simulink model "untitled2"  (R2022b)
settings: Solver=FixedStepAuto  StartTime=0  StopTime=1500  FixedStep=0.01  RelTol=1e-3
undefined symbols (not defined in the file or in its folder): sigbuilder_block
libraries: slpidlib x2
settings Model: Creator=hp  LastModifiedBy=hp

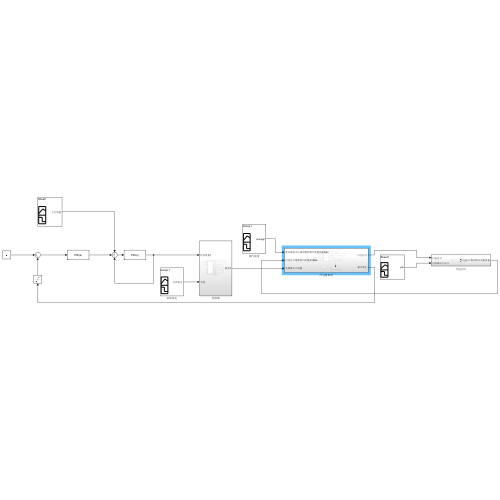
[thumbnail: Simulink's stored preview of the top-level diagram]
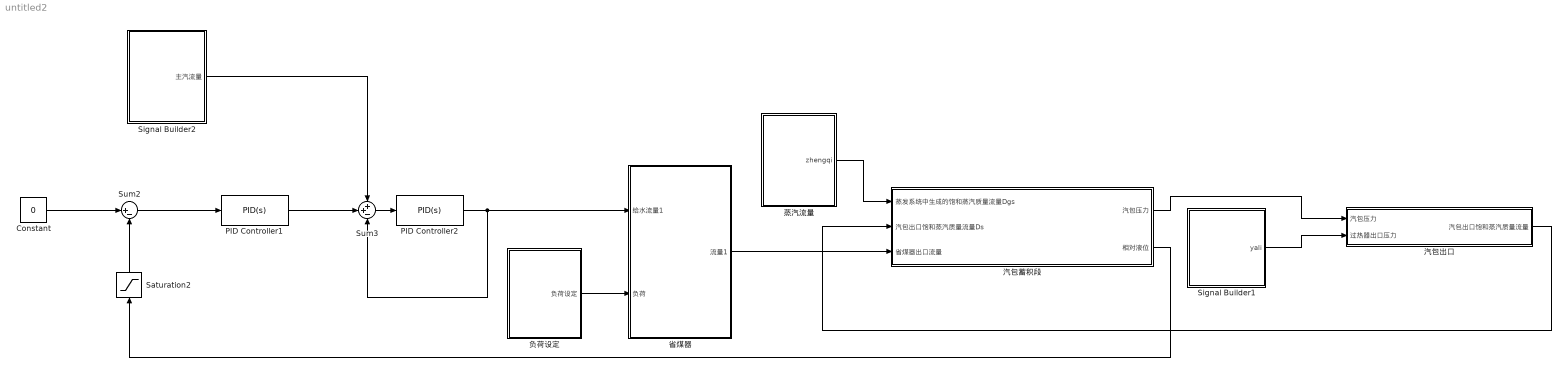
== system untitled2 ==
  Constant : Constant  Value=0
  PID Controller1 : slpidlib/PID Controller  Controller=PID  Form=Parallel  TimeDomain=Continuous-time  UseExternalTs=off  SampleTime=-1  IntegratorMethod=Forward Euler  FilterMethod=Forward Euler  ControllerParametersSource=internal  P=203.8263761763  I=22.4302136842899  UseKiTs=off  D=314.119346774621  N=0.810831032432681  UseFilter=on  TunerSelectOption=Transfer Function Based (PID Tuner App)  InitialConditionSource=internal  InitialConditionForIntegrator=0  InitialConditionForFilter=0  DifferentiatorICPrevScaledInput=0  ExternalReset=none  TrackingMode=off  Kt=1  LimitOutput=off  SatLimitsSource=internal  UpperSaturationLimit=inf  LowerSaturationLimit=-inf  LinearizeAsGain=on  AntiWindupMode=none  Kb=1  LimitIntegrator=off  UpperIntegratorSaturationLimit=inf  LowerIntegratorSaturationLimit=-inf  POutMin=[]  POutMax=[]  IOutMin=[]  IOutMax=[]  DOutMin=[]  DOutMax=[]  NOutMin=[]  NOutMax=[]  SumOutMin=[]  SumOutMax=[]  SaturationOutMin=[]  SaturationOutMax=[]  PParamMin=[]  PParamMax=[]  IParamMin=[]  IParamMax=[]  DParamMin=[]  DParamMax=[]  NParamMin=[]  NParamMax=[]  KbParamMin=[]  KbParamMax=[]  KtParamMin=[]  KtParamMax=[]  KbOutMin=[]  KbOutMax=[]  KtOutMin=[]  KtOutMax=[]  IntegratorOutMin=[]  IntegratorOutMax=[]  FilterOutMin=[]  FilterOutMax=[]  SumI1OutMin=[]  SumI1OutMax=[]  SumI2OutMin=[]  SumI2OutMax=[]  SumI3OutMin=[]  SumI3OutMax=[]  SumI4OutMin=[]  SumI4OutMax=[]  SumDOutMin=[]  SumDOutMax=[]  DifferentiatorOutMin=[]  DifferentiatorOutMax=[]  FilterDiffOutCoefMin=[]  FilterDiffOutCoefMax=[]  ReciprocalOutMin=[]  ReciprocalOutMax=[]  SumDenOutMin=[]  SumDenOutMax=[]  SumNumOutMin=[]  SumNumOutMax=[]  DivideOutMin=[]  DivideOutMax=[]  UdiffTsProdOutMin=[]  UdiffTsProdOutMax=[]  NTsProdOutMin=[]  NTsProdOutMax=[]  UintegralTsProdOutMin=[]  UintegralTsProdOutMax=[]  UngainTsProdOutMin=[]  UngainTsProdOutMax=[]  ClampingZeroOutDataTypeStr=Inherit: Inherit via back propagation  ClampingZeroOutMin=[]  ClampingZeroOutMax=[]  FilterDenConstantOutDataTypeStr=Inherit: Inherit via back propagation  FilterDenConstantOutMin=[]  FilterDenConstantOutMax=[]  PCopyOutDataTypeStr=Inherit: Inherit via back propagation  PCopyOutMin=[]  PCopyOutMax=[]  NCopyOutDataTypeStr=Inherit: Inherit via back propagation  NCopyOutMin=[]  NCopyOutMax=[]  IntegratorContinuousStateAttributes=''  IntegratorStateMustResolveToSignalObject=off  IntegratorRTWStateStorageClass=Auto  FilterContinuousStateAttributes=''  FilterStateMustResolveToSignalObject=off  FilterRTWStateStorageClass=Auto  ParallelPVariant=InternalParameters  IdealPVariant=Disabled  IVariant=InternalParameters  DVariant=InternalParameters  IntegratorVariant=Continuous  SatVariant=Disabled  AWVariant=Passthrough  PCopyVariant=Disabled  TRVariant=Disabled  FdbkBlocksVariant=Forward  IdealPFdbkVariant=Disabled  SatFdbkVariant=Disabled  DerivativeFilterVariant=ContFilter  NVariant=InternalParameters  NCopyVariant=Disabled  FilterICVariant=InternalICsFilter  IntegratorICVariant=InternalICs  ExternalResetVariant=Disabled  TRSumVariant=Passthrough  SumFdbkVariant=Disabled  SumVariant=Sum_PID  TsampFilterVariant=InternalTs  TsampNgainVariant=Passthrough  TsampIntegralVariant=Passthrough  ExternalSaturationOutDataTypeStr=Inherit: Same as second input
  PID Controller2 : slpidlib/PID Controller  Controller=PID  Form=Parallel  TimeDomain=Continuous-time  UseExternalTs=off  SampleTime=-1  IntegratorMethod=Forward Euler  FilterMethod=Forward Euler  ControllerParametersSource=internal  P=0.00527059631029743  I=1.6113586492284e-05  UseKiTs=off  D=0.389685831097133  N=0.0914334420746481  UseFilter=on  TunerSelectOption=Transfer Function Based (PID Tuner App)  InitialConditionSource=internal  InitialConditionForIntegrator=0  InitialConditionForFilter=0  DifferentiatorICPrevScaledInput=0  ExternalReset=none  TrackingMode=off  Kt=1  LimitOutput=off  SatLimitsSource=internal  UpperSaturationLimit=inf  LowerSaturationLimit=-inf  LinearizeAsGain=on  AntiWindupMode=none  Kb=1  LimitIntegrator=off  UpperIntegratorSaturationLimit=inf  LowerIntegratorSaturationLimit=-inf  POutMin=[]  POutMax=[]  IOutMin=[]  IOutMax=[]  DOutMin=[]  DOutMax=[]  NOutMin=[]  NOutMax=[]  SumOutMin=[]  SumOutMax=[]  SaturationOutMin=[]  SaturationOutMax=[]  PParamMin=[]  PParamMax=[]  IParamMin=[]  IParamMax=[]  DParamMin=[]  DParamMax=[]  NParamMin=[]  NParamMax=[]  KbParamMin=[]  KbParamMax=[]  KtParamMin=[]  KtParamMax=[]  KbOutMin=[]  KbOutMax=[]  KtOutMin=[]  KtOutMax=[]  IntegratorOutMin=[]  IntegratorOutMax=[]  FilterOutMin=[]  FilterOutMax=[]  SumI1OutMin=[]  SumI1OutMax=[]  SumI2OutMin=[]  SumI2OutMax=[]  SumI3OutMin=[]  SumI3OutMax=[]  SumI4OutMin=[]  SumI4OutMax=[]  SumDOutMin=[]  SumDOutMax=[]  DifferentiatorOutMin=[]  DifferentiatorOutMax=[]  FilterDiffOutCoefMin=[]  FilterDiffOutCoefMax=[]  ReciprocalOutMin=[]  ReciprocalOutMax=[]  SumDenOutMin=[]  SumDenOutMax=[]  SumNumOutMin=[]  SumNumOutMax=[]  DivideOutMin=[]  DivideOutMax=[]  UdiffTsProdOutMin=[]  UdiffTsProdOutMax=[]  NTsProdOutMin=[]  NTsProdOutMax=[]  UintegralTsProdOutMin=[]  UintegralTsProdOutMax=[]  UngainTsProdOutMin=[]  UngainTsProdOutMax=[]  ClampingZeroOutDataTypeStr=Inherit: Inherit via back propagation  ClampingZeroOutMin=[]  ClampingZeroOutMax=[]  FilterDenConstantOutDataTypeStr=Inherit: Inherit via back propagation  FilterDenConstantOutMin=[]  FilterDenConstantOutMax=[]  PCopyOutDataTypeStr=Inherit: Inherit via back propagation  PCopyOutMin=[]  PCopyOutMax=[]  NCopyOutDataTypeStr=Inherit: Inherit via back propagation  NCopyOutMin=[]  NCopyOutMax=[]  IntegratorContinuousStateAttributes=''  IntegratorStateMustResolveToSignalObject=off  IntegratorRTWStateStorageClass=Auto  FilterContinuousStateAttributes=''  FilterStateMustResolveToSignalObject=off  FilterRTWStateStorageClass=Auto  ParallelPVariant=InternalParameters  IdealPVariant=Disabled  IVariant=InternalParameters  DVariant=InternalParameters  IntegratorVariant=Continuous  SatVariant=Disabled  AWVariant=Passthrough  PCopyVariant=Disabled  TRVariant=Disabled  FdbkBlocksVariant=Forward  IdealPFdbkVariant=Disabled  SatFdbkVariant=Disabled  DerivativeFilterVariant=ContFilter  NVariant=InternalParameters  NCopyVariant=Disabled  FilterICVariant=InternalICsFilter  IntegratorICVariant=InternalICs  ExternalResetVariant=Disabled  TRSumVariant=Passthrough  SumFdbkVariant=Disabled  SumVariant=Sum_PID  TsampFilterVariant=InternalTs  TsampNgainVariant=Passthrough  TsampIntegralVariant=Passthrough  ExternalSaturationOutDataTypeStr=Inherit: Same as second input
  Saturation2 : Saturate  UpperLimit=50  LowerLimit=-50
  Signal Builder1 : Subsystem  Tag=STV Subsys  LoadFcn=sigbuilder_block('load');  StartFcn=sigbuilder_block('start');  StopFcn=sigbuilder_block('stop');  ClipboardFcn=sigbuilder_block('clipboard');  mask(Sigbuilder block){tuvar=[0:10]}
      mask help: Simulink:masks:SigbuilderBlock_MD
      mask init:
      | if ~strcmp(get_param(bdroot(gcbh),'SimulationStatus'),'stopped') tuvar = sigbuilder_block('maskInit'); end
      settings: CopyFcn=sigbuilder_block('copy');  DeleteFcn=sigbuilder_block('delete');  ModelCloseFcn=sigbuilder_block('modelClose');  PreSaveFcn=sigbuilder_block('preSave');  PauseFcn=sigbuilder_block('pause');  ContinueFcn=sigbuilder_block('continue');  NameChangeFcn=sigbuilder_block('namechange');  OpenFcn=sigbuilder_block('open',[430.8 150 550.8 400.2 ]);  CloseFcn=sigbuilder_block('close');
      mask Display: plot(0, 0, 100, 100,[2, 2, 32, 32, 2], [68, 8, 8, 68, 68],[32, 2], [38, 38], [32, 19, 2],[53, 60, 44], [32, 17, 17, 2],[16, 16, 31, 31]);txt = getActiveGroup(gcbh);text(2, 100, txt,'verticalAlignment', 'top');
  Signal Builder2 : Subsystem  Tag=STV Subsys  LoadFcn=sigbuilder_block('load');  StartFcn=sigbuilder_block('start');  StopFcn=sigbuilder_block('stop');  ClipboardFcn=sigbuilder_block('clipboard');  mask(Sigbuilder block){tuvar=[0:10]}
      mask help: Simulink:masks:SigbuilderBlock_MD
      mask init:
      | if ~strcmp(get_param(bdroot(gcbh),'SimulationStatus'),'stopped') tuvar = sigbuilder_block('maskInit'); end
      settings: CopyFcn=sigbuilder_block('copy');  DeleteFcn=sigbuilder_block('delete');  ModelCloseFcn=sigbuilder_block('modelClose');  PreSaveFcn=sigbuilder_block('preSave');  PauseFcn=sigbuilder_block('pause');  ContinueFcn=sigbuilder_block('continue');  NameChangeFcn=sigbuilder_block('namechange');  OpenFcn=sigbuilder_block('open',[0.6 30.6 574.8 556.2 ]);  CloseFcn=sigbuilder_block('close');
      mask Display: plot(0, 0, 100, 100,[2, 2, 32, 32, 2], [68, 8, 8, 68, 68],[32, 2], [38, 38], [32, 19, 2],[53, 60, 44], [32, 17, 17, 2],[16, 16, 31, 31]);txt = getActiveGroup(gcbh);text(2, 100, txt,'verticalAlignment', 'top');
  Sum2 : Sum  Inputs=|+-
  Sum3 : Sum  Inputs=++-
  汽包出口 : Subsystem
  汽包蓄积段 : Subsystem
  省煤器 : Subsystem
  蒸汽流量 : Subsystem  Tag=STV Subsys  LoadFcn=sigbuilder_block('load');  StartFcn=sigbuilder_block('start');  StopFcn=sigbuilder_block('stop');  ClipboardFcn=sigbuilder_block('clipboard');  mask(Sigbuilder block){tuvar=[0:10]}
      mask help: Simulink:masks:SigbuilderBlock_MD
      mask init:
      | if ~strcmp(get_param(bdroot(gcbh),'SimulationStatus'),'stopped') tuvar = sigbuilder_block('maskInit'); end
      settings: CopyFcn=sigbuilder_block('copy');  DeleteFcn=sigbuilder_block('delete');  ModelCloseFcn=sigbuilder_block('modelClose');  PreSaveFcn=sigbuilder_block('preSave');  PauseFcn=sigbuilder_block('pause');  ContinueFcn=sigbuilder_block('continue');  NameChangeFcn=sigbuilder_block('namechange');  OpenFcn=sigbuilder_block('open',[5.4 5.4 1141.2 581.4 ]);  CloseFcn=sigbuilder_block('close');
      mask Display: plot(0, 0, 100, 100,[2, 2, 32, 32, 2], [68, 8, 8, 68, 68],[32, 2], [38, 38], [32, 19, 2],[53, 60, 44], [32, 17, 17, 2],[16, 16, 31, 31]);txt = getActiveGroup(gcbh);text(2, 100, txt,'verticalAlignment', 'top');
  负荷设定 : Subsystem  Tag=STV Subsys  LoadFcn=sigbuilder_block('load');  StartFcn=sigbuilder_block('start');  StopFcn=sigbuilder_block('stop');  ClipboardFcn=sigbuilder_block('clipboard');  mask(Sigbuilder block){tuvar=[0:10]}
      mask help: Simulink:masks:SigbuilderBlock_MD
      mask init:
      | if ~strcmp(get_param(bdroot(gcbh),'SimulationStatus'),'stopped') tuvar = sigbuilder_block('maskInit'); end
      settings: CopyFcn=sigbuilder_block('copy');  DeleteFcn=sigbuilder_block('delete');  ModelCloseFcn=sigbuilder_block('modelClose');  PreSaveFcn=sigbuilder_block('preSave');  PauseFcn=sigbuilder_block('pause');  ContinueFcn=sigbuilder_block('continue');  NameChangeFcn=sigbuilder_block('namechange');  OpenFcn=sigbuilder_block('open',[5.4 5.4 1141.2 581.4 ]);  CloseFcn=sigbuilder_block('close');
      mask Display: plot(0, 0, 100, 100,[2, 2, 32, 32, 2], [68, 8, 8, 68, 68],[32, 2], [38, 38], [32, 19, 2],[53, 60, 44], [32, 17, 17, 2],[16, 16, 31, 31]);txt = getActiveGroup(gcbh);text(2, 100, txt,'verticalAlignment', 'top');
  wires:
  Signal Builder1/1(yali) -> 汽包出口/2(过热器出口压力)
  汽包出口/1(汽包出口饱和蒸汽质量流量) -> 汽包蓄积段/2(汽包出口饱和蒸汽质量流量Ds)
  汽包蓄积段/1(汽包压力) -> 汽包出口/1(汽包压力)
  Saturation2/1 -> Sum2/2
  Constant/1 -> Sum2/1
  Sum2/1 -> PID Controller1/1
  PID Controller1/1 -> Sum3/2
  PID Controller2/1 -> Sum3/3, 省煤器/1(给水流量1)
  汽包蓄积段/2(相对液位) -> Saturation2/1
  Sum3/1 -> PID Controller2/1
  省煤器/1(流量1) -> 汽包蓄积段/3(省煤器出口流量)
  蒸汽流量/1(zhengqi) -> 汽包蓄积段/1(蒸发系统中生成的饱和蒸汽质量流量Dgs)
  Signal Builder2/1(主汽流量) -> Sum3/1
  负荷设定/1(负荷设定) -> 省煤器/2(负荷)

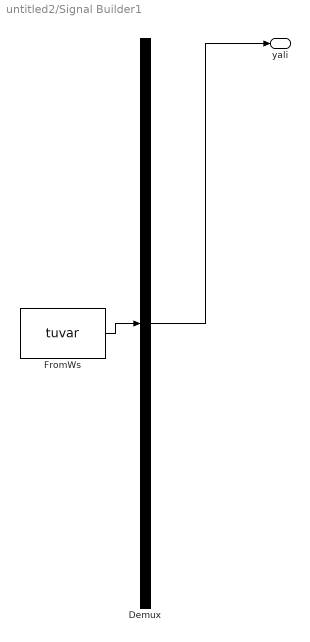
== system untitled2/Signal Builder1 ==
  Demux : Demux  Tag=STV Demux  Outputs=1
      settings: DisplayOption=none
  FromWs : FromWorkspace  Tag=STV FromWs  VariableName=tuvar
      SigBuilderData=|
      | common.afterFinalStr = 'Extrapolate'
      | common.sampleTime = 0
      | dataSet.timeRange = [0 1500]
      | dataSet.name = 'Sheet1'
      | sbobj.Groups.Name = 'Sheet1'
      | sbobj.Groups.Signals.Name = 'yali'
      | sbobj.Groups.Signals.XData = [0 5 10 15 20 25 30 35 40 45 50 55 60 65 70 75 80 85 90 95 100 105 110 115 120 125 130 135 140 145 150 155 160 165 170 175 180 185 190 195 200 205 210 215 220 225 230 235 240 245 250 255 260 265 270 275 280 285 290 295 300 305 310 315 320 325 330 335 340 345 350 355 360 365 370 375 380 385 390 395 400 405 410 415 420 425 430 435 440 445 450 455 460 465 470 475 480 485 490 495 500 505 510 515 520 525 530 535 540 545 550 555 560 565 570 575 580 585 590 595 600 605 610 615 620 625 630 635 640 645 650 655 660 665 670 675 680 685 690 695 700 705 710 715 720 725 730 735 740 745 750 755 760 765 770 775 780 785 790 795 800 805 810 815 820 825 830 835 840 845 850 855 860 865 870 875 880 885 890 895 900 905 910 915 920 925 930 935 940 945 950 955 960 965 970 975 980 985 990 995 1000 1005 1010 1015 1020 1025 1030 1035 1040 1045 1050 1055 1060 1065 1070 1075 1080 1085 1090 1095 1100 1105 1110 1115 1120 1125 1130 1135 1140 1145 1150 1155 1160 1165 1170 1175 1180 1185 1190 1195 1200 1205 1210 1215 1220 1225 1230 1235 1240 1245 1250 1255 1260 1265 1270 1275 1280 1285 1290 1295 1300 1305 1310 1315 1320 1325 1330 1335 1340 1345 1350 1355 1360 1365 1370 1375 1380 1385 1390 1395 1400 1405 1410 1415 1420 1425 1430 1435 1440 1445 1450 1455 1460 1465 1470 1475 1480 1485 1490 1495 1500]
      | sbobj.Groups.Signals.YData = [10 13.4582 13.396 13.3935 13.5342 13.7027 13.851 13.9729 14.2031 14.4422 14.6355 14.8136 ... (301 elements, 1x301)]
      | sbobj.Groups.TimeRange = [0 1500]
  yali : Outport  Tag=STV Outport
  wires:
  Demux/1 -> yali/1
  FromWs/1 -> Demux/1

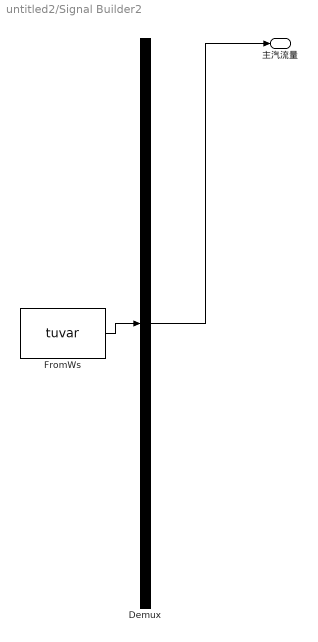
== system untitled2/Signal Builder2 ==
  Demux : Demux  Tag=STV Demux  Outputs=1
      settings: DisplayOption=none
  FromWs : FromWorkspace  Tag=STV FromWs  VariableName=tuvar
      SigBuilderData=|
      | common.afterFinalStr = 'Extrapolate'
      | common.sampleTime = 0
      | dataSet.timeRange = [0 1500]
      | dataSet.name = 'Sheet1'
      | sbobj.Groups.Name = 'Sheet1'
      | sbobj.Groups.Signals.Name = '主汽流量'
      | sbobj.Groups.Signals.XData = [0 5 10 15 20 25 30 35 40 45 50 55 60 65 70 75 80 85 90 95 100 105 110 115 120 125 130 135 140 145 150 155 160 165 170 175 180 185 190 195 200 205 210 215 220 225 230 235 240 245 250 255 260 265 270 275 280 285 290 295 300 305 310 315 320 325 330 335 340 345 350 355 360 365 370 375 380 385 390 395 400 405 410 415 420 425 430 435 440 445 450 455 460 465 470 475 480 485 490 495 500 505 510 515 520 525 530 535 540 545 550 555 560 565 570 575 580 585 590 595 600 605 610 615 620 625 630 635 640 645 650 655 660 665 670 675 680 685 690 695 700 705 710 715 720 725 730 735 740 745 750 755 760 765 770 775 780 785 790 795 800 805 810 815 820 825 830 835 840 845 850 855 860 865 870 875 880 885 890 895 900 905 910 915 920 925 930 935 940 945 950 955 960 965 970 975 980 985 990 995 1000 1005 1010 1015 1020 1025 1030 1035 1040 1045 1050 1055 1060 1065 1070 1075 1080 1085 1090 1095 1100 1105 1110 1115 1120 1125 1130 1135 1140 1145 1150 1155 1160 1165 1170 1175 1180 1185 1190 1195 1200 1205 1210 1215 1220 1225 1230 1235 1240 1245 1250 1255 1260 1265 1270 1275 1280 1285 1290 1295 1300 1305 1310 1315 1320 1325 1330 1335 1340 1345 1350 1355 1360 1365 1370 1375 1380 1385 1390 1395 1400 1405 1410 1415 1420 1425 1430 1435 1440 1445 1450 1455 1460 1465 1470 1475 1480 1485 1490 1495 1500]
      | sbobj.Groups.Signals.YData = [0 398.482 345.4859 388.8564 416.7382 419.4128 415.3315 410.8408 389.3783 389.3634 390.9978 392.5043 ... (301 elements, 1x301)]
      | sbobj.Groups.TimeRange = [0 1500]
  主汽流量 : Outport  Tag=STV Outport
  wires:
  Demux/1 -> 主汽流量/1
  FromWs/1 -> Demux/1

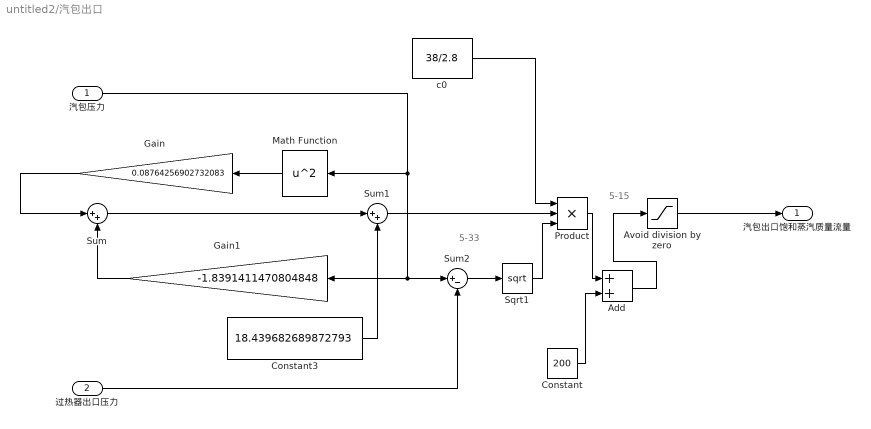
== system untitled2/汽包出口 ==
  note: 5-15
  note: 5-33
  汽包压力 : Inport
  过热器出口压力 : Inport  Port=2
  Add : Sum
  Avoid division by zero : Saturate  UpperLimit=600  LowerLimit=100
  Constant : Constant  Value=200
  Constant3 : Constant  Value=18.439682689872793
  Gain : Gain  Gain=0.08764256902732083
  Gain1 : Gain  Gain=-1.8391411470804848
  Math Function : Math  Operator=square  SignedPower=on
  Product : Product  Inputs=3
  Sqrt1 : Sqrt
  Sum : Sum  Inputs=|++
  Sum1 : Sum  Inputs=|++
  Sum2 : Sum  Inputs=|+-
  c0 : Constant  Value=38/2.8
  汽包出口饱和蒸汽质量流量 : Outport
  wires:
  Sum2/1 -> Sqrt1/1
  Gain/1 -> Sum/1
  Sum1/1 -> Product/2
  Constant/1 -> Add/2
  汽包压力/1 -> Sum2/1, Gain1/1, Math Function/1
  Add/1 -> Avoid division by zero/1
  c0/1 -> Product/1
  Product/1 -> Add/1
  Math Function/1 -> Gain/1
  Sqrt1/1 -> Product/3
  Avoid division by zero/1 -> 汽包出口饱和蒸汽质量流量/1
  Gain1/1 -> Sum/2
  过热器出口压力/1 -> Sum2/2
  Constant3/1 -> Sum1/2
  Sum/1 -> Sum1/1

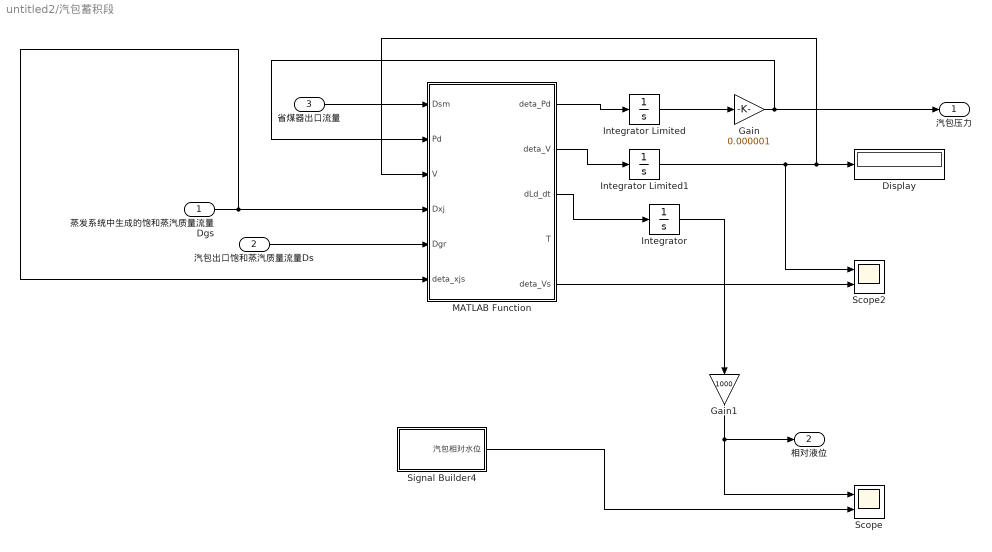
== system untitled2/汽包蓄积段 ==
  蒸发系统中生成的饱和蒸汽质量流量Dgs : Inport
  汽包出口饱和蒸汽质量流量Ds : Inport  Port=2
  省煤器出口流量 : Inport  Port=3
  Display : Display
  Gain : Gain  Gain=0.000001
  Gain1 : Gain  Gain=1000
  Integrator : Integrator
  Integrator Limited : Integrator  InitialCondition=18000000  LimitOutput=on  UpperSaturationLimit=30000000  LowerSaturationLimit=6000000
  Integrator Limited1 : Integrator  InitialCondition=50  LimitOutput=on  UpperSaturationLimit=225  LowerSaturationLimit=0
  MATLAB Function : MATLAB Function  TreatAsAtomicUnit=on
  Scope : Scope  NumInputPorts=2
  Scope2 : Scope  NumInputPorts=2
  Signal Builder4 : Subsystem  Tag=STV Subsys  LoadFcn=sigbuilder_block('load');  StartFcn=sigbuilder_block('start');  StopFcn=sigbuilder_block('stop');  ClipboardFcn=sigbuilder_block('clipboard');  mask(Sigbuilder block){tuvar=[0:10]}
      mask help: Simulink:masks:SigbuilderBlock_MD
      mask init:
      | if ~strcmp(get_param(bdroot(gcbh),'SimulationStatus'),'stopped') tuvar = sigbuilder_block('maskInit'); end
      settings: CopyFcn=sigbuilder_block('copy');  DeleteFcn=sigbuilder_block('delete');  ModelCloseFcn=sigbuilder_block('modelClose');  PreSaveFcn=sigbuilder_block('preSave');  PauseFcn=sigbuilder_block('pause');  ContinueFcn=sigbuilder_block('continue');  NameChangeFcn=sigbuilder_block('namechange');  OpenFcn=sigbuilder_block('open',[5.4 5.4 1141.2 581.4 ]);  CloseFcn=sigbuilder_block('close');
      mask Display: plot(0, 0, 100, 100,[2, 2, 32, 32, 2], [68, 8, 8, 68, 68],[32, 2], [38, 38], [32, 19, 2],[53, 60, 44], [32, 17, 17, 2],[16, 16, 31, 31]);txt = getActiveGroup(gcbh);text(2, 100, txt,'verticalAlignment', 'top');
  汽包压力 : Outport
  相对液位 : Outport  Port=2
  wires:
  Integrator Limited1/1 -> MATLAB Function/3(V), Display/1, Scope2/1
  Integrator/1 -> Gain1/1
  蒸发系统中生成的饱和蒸汽质量流量Dgs/1 -> MATLAB Function/6(deta_xjs), MATLAB Function/4(Dxj)
  汽包出口饱和蒸汽质量流量Ds/1 -> MATLAB Function/5(Dgr)
  省煤器出口流量/1 -> MATLAB Function/1(Dsm)
  Gain/1 -> MATLAB Function/2(Pd), 汽包压力/1
  Gain1/1 -> Scope/1, 相对液位/1
  MATLAB Function/1(deta_Pd) -> Integrator Limited/1
  MATLAB Function/3(dLd_dt) -> Integrator/1
  Integrator Limited/1 -> Gain/1
  MATLAB Function/2(deta_V) -> Integrator Limited1/1
  MATLAB Function/5(deta_Vs) -> Scope2/2
  Signal Builder4/1(汽包相对水位) -> Scope/2

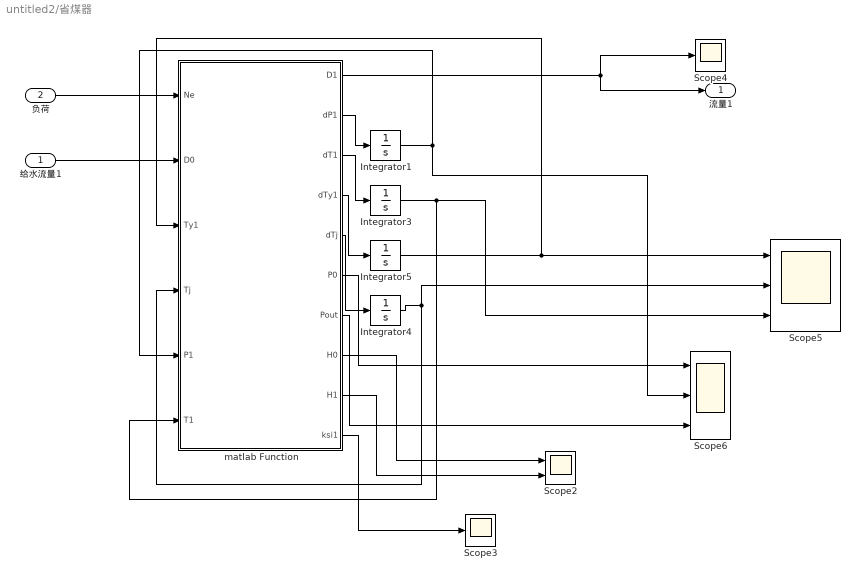
== system untitled2/省煤器 ==
  给水流量1 : Inport
  负荷 : Inport  Port=2
  Integrator1 : Integrator  InitialCondition=18.5
  Integrator3 : Integrator  InitialCondition=300  LimitOutput=on  UpperSaturationLimit=1000  LowerSaturationLimit=1
  Integrator4 : Integrator  InitialCondition=300  LimitOutput=on  UpperSaturationLimit=10000  LowerSaturationLimit=10
  Integrator5 : Integrator  InitialCondition=482  LimitOutput=on  UpperSaturationLimit=2000  LowerSaturationLimit=1
  Scope2 : Scope  NumInputPorts=2
  Scope3 : Scope
  Scope4 : Scope
  Scope5 : Scope  NumInputPorts=3
  Scope6 : Scope  NumInputPorts=3
  matlab Function : MATLAB Function  TreatAsAtomicUnit=on
  流量1 : Outport
  wires:
  matlab Function/9(H1) -> Scope2/2
  matlab Function/8(H0) -> Scope2/1
  Integrator4/1 -> matlab Function/4(Tj), Scope5/2
  matlab Function/10(ksi1) -> Scope3/1
  负荷/1 -> matlab Function/1(Ne)
  matlab Function/6(P0) -> Scope6/1
  matlab Function/5(dTj) -> Integrator4/1
  matlab Function/3(dT1) -> Integrator3/1
  matlab Function/7(Pout) -> Scope6/3
  Integrator3/1 -> Scope5/3, matlab Function/6(T1)
  matlab Function/1(D1) -> 流量1/1, Scope4/1
  matlab Function/4(dTy1) -> Integrator5/1
  Integrator5/1 -> matlab Function/3(Ty1), Scope5/1
  Integrator1/1 -> matlab Function/5(P1), Scope6/2
  matlab Function/2(dP1) -> Integrator1/1
  给水流量1/1 -> matlab Function/2(D0)

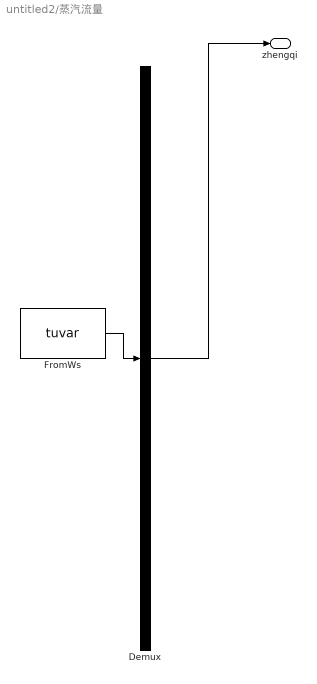
== system untitled2/蒸汽流量 ==
  Demux : Demux  Tag=STV Demux  Outputs=1
      settings: DisplayOption=none
  FromWs : FromWorkspace  Tag=STV FromWs  VariableName=tuvar
      SigBuilderData=|
      | common.afterFinalStr = 'Extrapolate'
      | common.sampleTime = 0
      | dataSet.timeRange = [0 1500]
      | dataSet.name = 'Group 1'
      | sbobj.Groups.Name = 'Group 1'
      | sbobj.Groups.Signals.Name = 'zhengqi'
      | sbobj.Groups.Signals.XData = [0 5 10 15 20 25 30 35 40 45 50 55 60 65 70 75 80 85 90 95 100 105 110 115 120 125 130 135 140 145 150 155 160 165 170 175 180 185 190 195 200 205 210 215 220 225 230 235 240 245 250 255 260 265 270 275 280 285 290 295 300 305 310 315 320 325 330 335 340 345 350 355 360 365 370 375 380 385 390 395 400 405 410 415 420 425 430 435 440 445 450 455 460 465 470 475 480 485 490 495 500 505 510 515 520 525 530 535 540 545 550 555 560 565 570 575 580 585 590 595 600 605 610 615 620 625 630 635 640 645 650 655 660 665 670 675 680 685 690 695 700 705 710 715 720 725 730 735 740 745 750 755 760 765 770 775 780 785 790 795 800 805 810 815 820 825 830 835 840 845 850 855 860 865 870 875 880 885 890 895 900 905 910 915 920 925 930 935 940 945 950 955 960 965 970 975 980 985 990 995 1000 1005 1010 1015 1020 1025 1030 1035 1040 1045 1050 1055 1060 1065 1070 1075 1080 1085 1090 1095 1100 1105 1110 1115 1120 1125 1130 1135 1140 1145 1150 1155 1160 1165 1170 1175 1180 1185 1190 1195 1200 1205 1210 1215 1220 1225 1230 1235 1240 1245 1250 1255 1260 1265 1270 1275 1280 1285 1290 1295 1300 1305 1310 1315 1320 1325 1330 1335 1340 1345 1350 1355 1360 1365 1370 1375 1380 1385 1390 1395 1400 1405 1410 1415 1420 1425 1430 1435 1440 1445 1450 1455 1460 1465 1470 1475 1480 1485 1490 1495 1500]
      | sbobj.Groups.Signals.YData = [100 107.95 376.72 521.32 468.69 436.83 424.31 417.72 419.87 423.04 424.17 424.51 ... (301 elements, 1x301)]
      | sbobj.Groups.TimeRange = [0 1500]
  zhengqi : Outport  Tag=STV Outport
  wires:
  FromWs/1 -> Demux/1
  Demux/1 -> zhengqi/1

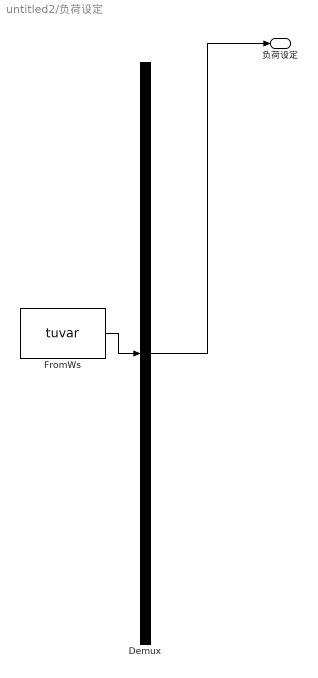
== system untitled2/负荷设定 ==
  Demux : Demux  Tag=STV Demux  Outputs=1
      settings: DisplayOption=none
  FromWs : FromWorkspace  Tag=STV FromWs  VariableName=tuvar
      SigBuilderData=|
      | common.afterFinalStr = 'Extrapolate'
      | common.sampleTime = 0
      | dataSet.timeRange = [1 518400]
      | dataSet.name = 'Group 1'
      | sbobj.Groups.Name = 'Group 1'
      | sbobj.Groups.Signals.Name = '负荷设定'
      | sbobj.Groups.Signals.XData = [1 2 3 4 5 6 7 8 9 10 11 12 ... (518400 elements, 1x518400)]
      | sbobj.Groups.Signals.YData = [447.476196289 447.476196289 447.476196289 447.476196289 447.476196289 447.476196289 447.476196289 447.476196289 447.476196289 447.476196289 447.476196289 447.476196289 ... (518400 elements, 1x518400)]
      | sbobj.Groups.TimeRange = [1 518400]
  负荷设定 : Outport  Tag=STV Outport
  wires:
  FromWs/1 -> Demux/1
  Demux/1 -> 负荷设定/1

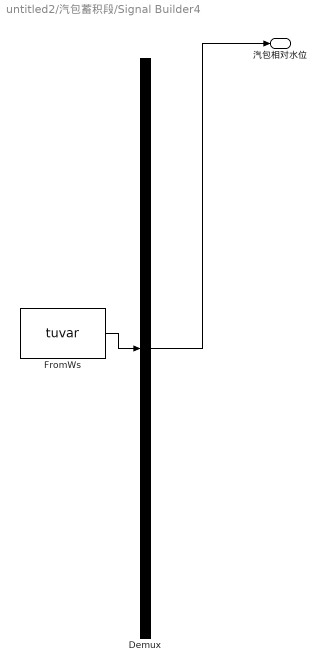
== system untitled2/汽包蓄积段/Signal Builder4 ==
  Demux : Demux  Tag=STV Demux  Outputs=1
      settings: DisplayOption=none
  FromWs : FromWorkspace  Tag=STV FromWs  VariableName=tuvar
      SigBuilderData=|
      | common.afterFinalStr = 'Extrapolate'
      | common.sampleTime = 0
      | dataSet.timeRange = [0 518400]
      | dataSet.name = 'Group 1'
      | sbobj.Groups.Name = 'Group 1'
      | sbobj.Groups.Signals.Name = '汽包相对水位'
      | sbobj.Groups.Signals.XData = [0 2 3 4 5 6 7 8 9 10 11 12 ... (518400 elements, 1x518400)]
      | sbobj.Groups.Signals.YData = [24.8626384735 24.8626384735 24.8626384735 18.124917984 18.124917984 18.124917984 11.550860405 11.550860405 11.550860405 11.550860405 11.550860405 4.94502353668 ... (518400 elements, 1x518400)]
      | sbobj.Groups.TimeRange = [0 518400]
  汽包相对水位 : Outport  Tag=STV Outport
  wires:
  FromWs/1 -> Demux/1
  Demux/1 -> 汽包相对水位/1

== matlab function untitled2/汽包蓄积段/MATLAB Function ==
  data: Dsm input; deta_Pd output; Pd input; V input; Dxj input; Dgr input; deta_xjs input; deta_V output; dLd_dt output; T output; deta_Vs output
function [deta_Pd,deta_V,dLd_dt,T,deta_Vs]= fcn(Dsm,Pd,V,Dxj,Dgr,deta_xjs)
coder.extrinsic('XSteam');
coder.extrinsic('IAPWS_IF97');
rho=0;rhos=0;T=0;
R=461.5;%蒸汽气体常数
Vqb=256;%汽包
rho=XSteam('rhoL_p',10*Pd);%液体密度
rhos=XSteam('rhoV_p',10*Pd);%蒸汽密度
T=XSteam('Tsat_p',Pd*10);
deta_V=(Dsm-Dxj)/rho;%Vw流体的体积变化
deta_Vs=(Dxj-deta_xjs)/rhos;%蒸汽体积的变化
deta_Pd=R*(T+273.15)/(Vqb-V)*(Dxj-Dgr);%压力变化相关的量
Ad=45.318;
dLd_dt=1/Ad*(deta_V+deta_Vs);

== matlab function untitled2/省煤器/matlab Function ==
  data: D1 output size=1; dP1 output size=1; dT1 output size=1; dTy1 output size=1; Ne input size=1; D0 input; Ty1 input; Tj input; dTj output; P1 input; T1 input; P0 output; Pout output; H0 output; H1 output; ksi1 output
function [D1, dP1, dT1, dTy1,dTj,P0,Pout,H0,H1,ksi1]  = fcn(Ne, D0, Ty1,Tj,P1,T1)
    Mj = 5000;
    cj = 0.5;
    V =  80;
    Vy = 100;
    ky = 80;
    
  
   P0=[-4.9635549e-8,6.63318631e-5,-0.0153,15.5287]*[Ne^3,Ne^2, Ne, 1]';
    T0=  [-5.552223890598186e-5,0.188222106275285,187.4638;]*[Ne^2, Ne, 1]'; %拟合,后续要算H0
   


    Ty0=  [-0.00024444444444444345,0.4033333333333324,350.0000000000002;]*[Ne^2, Ne, 1]'; %拟合，算dTy1
    

    
    mid1 = [-0.0015650666666666663,2.424473333333333,-357.2819999999998;
         -1.6666666664670333e-09,1.4033333331143116e-06,-3.699999995103936e-05;
          -0.00018639250135555523,0.16768895880333307, -29.693576604999947]*[Ne^2,Ne, 1]';

    Dy = 0.85*mid1(1); %算dTj和dTy1   
    ksi1 =20*mid1(2);%算D1要用的，输出有的 
    kc =12*mid1(3);%算dT1与dTj的

    mid2 = [1210.86211811911,-1.59793418318532,-35.8884167229680,0.313417735621854,-0.000455489263743170,-0.867613946591206,0.00280501652204646,-0.000615644347189089;
           -35.8884167229680,0.313417735621854,-0.867613946591206*2,2*0.00280501652204646,-0.000615644347189089,0,0,0
           ]*[1, T1, P1, P1*T1, T1^2, P1^2, P1^2*T1, P1*T1^2]';
    
    rho1 = mid2(1);%算D1与dT1的
    drho1 = mid2(2);%算dP1

    H0 =106.780612309849+3.54538497629407*T0-16.088116133118092*P0+0.063459069518316*P0*T0+0.001505531044285*T0^2+1.264454190598599*P0^2-0.007735643634244*P0^2*T0+1.086607348530378e-05*P0^2*T0^2; % 算dT1的   

    mid3=[2.91894501846895,4.48997695937590,-47.8864910940965,0.152989961918212,0.000109879475056696,6.18027726004829,-0.0348478482739920,4.78907792762745e-05;
        4.48997695937590,2*0.000109879475056696,0.152989961918212,0,0,-0.0348478482739920,2*4.78907792762745e-05,0]*[1, T1, P1, P1*T1, T1^2, P1^2, P1^2*T1, P1^2*T1^2]';

    H1 = mid3(1);%算dT1
    dHT1 = mid3(2);%算dT1

    dHP1 = [-47.8864910940965,0.152989961918212,2*6.18027726004829,-2*0.0348478482739920,2*4.78907792762745e-05;]*[1, T1, P1, P1*T1, P1*T1^2]'; % 算dT1  
   
    rhoy1 = [1.799999999999994e-05, -0.015979999999999953, 4.03699999999999;]*[Ty1^2, Ty1, 1]';%拟合    

    mid4=[-1.9999999999988916e-07, 0.0004899999999999016,0.9900000000000216;
          2.2204460486140494e-20,-0.0009200000000000152,0.8930000000000026;]*[Ty1^2, Ty1, 1]';%用物性表拟合    
    cy0 = mid4(1);% 算dTy1
    cy1 = mid4(2);%算 dTy1

    Pout=[2.85195241345460e-05	-0.0113109873432667	15.9447132979074]*[Ne^2,Ne, 1]';%算D1
    D1 = real(power(complex(rho1*(P1-Pout)/ksi1),0.5));

    
    dP1 = (D0-D1)/(V*drho1);
    dT1 = (D0*(H0-H1)+kc*real(power(complex(D1),0.8))*(Tj-T1)-V*rho1*dHP1*dP1)/(V*rho1*dHT1);
    dTj = (ky*real(power(complex(Dy),0.8))*(Ty1-Tj)-kc*real(power(complex(D1),0.8))*(Tj-T1))/(Mj*cj);
    dTy1 = (Dy*cy0*Ty0-Dy*cy1*Ty1-ky*real(power(complex(Dy),0.8))*(Ty1-Tj))/(rhoy1*Vy*cy1);
